simulink model "ex7_pitch"  (R2021b)
settings: Solver=FixedStepAuto  StartTime=0.0  StopTime=120  FixedStep=0.05  RelTol=1e-7
settings Model: Creator=steven  LastModifiedBy=steven

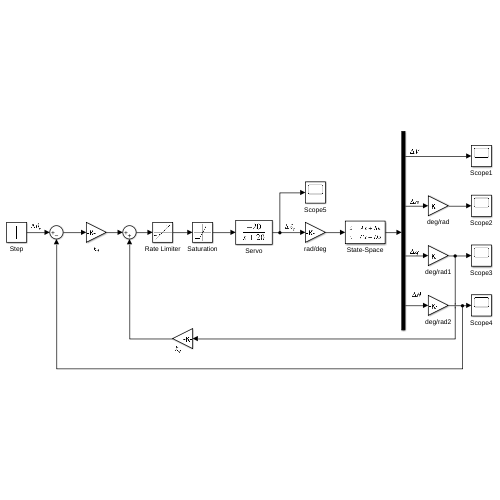
[thumbnail: Simulink's stored preview of the top-level diagram]
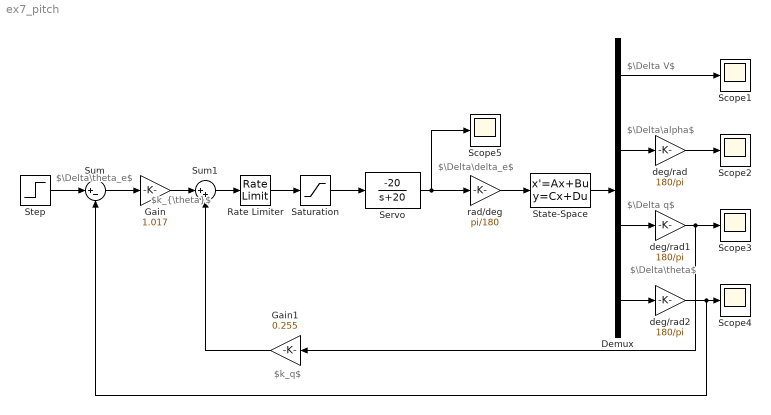
== system ex7_pitch ==
  note: $\Delta\alpha$
  note: $\Delta V$
  note: $\Delta q$
  note: $\Delta\theta$
  note: $\Delta\delta_e$
  note: $\Delta\theta_e$
  note: $k_{\theta}$
  note: $k_q$
  Demux : Demux
  Gain : Gain  Gain=1.017
  Gain1 : Gain  Gain=0.255
  Rate Limiter : RateLimiter  RisingSlewLimit=30  FallingSlewLimit=-30  SampleTimeMode=inherited
  Saturation : Saturate  UpperLimit=15  LowerLimit=-25
  Scope{1..5} (5 alike) : Scope
  Servo : TransferFcn  Numerator=[-20]  Denominator=[1 20]
  State-Space : StateSpace  A=[-0.0045,1.93,0,-9.8; -0.007, -2.02, 1, 0; 0.0062,-6.97,-2.948,0; 0,0,1,0]  B=[0;-0.16;-11.87;0]  C=eye(4)  D=[0;0;0;0]  InitialCondition=0
  Step : Step  Time=0  After=5  SampleTime=0  ZeroCross=off
  Sum : Sum  Inputs=|+-
  Sum1 : Sum  Inputs=|++
  deg/rad : Gain  Gain=180/pi
  deg/rad1 : Gain  Gain=180/pi
  deg/rad2 : Gain  Gain=180/pi
  rad/deg : Gain  Gain=pi/180
  wires:
  Step/1 -> Sum/1
  Saturation/1 -> Servo/1
  Gain/1 -> Sum1/1
  Sum1/1 -> Rate Limiter/1
  Sum/1 -> Gain/1
  Rate Limiter/1 -> Saturation/1
  Servo/1 -> Scope5/1, rad/deg/1
  rad/deg/1 -> State-Space/1
  State-Space/1 -> Demux/1
  Demux/2 -> deg/rad/1
  Demux/3 -> deg/rad1/1
  Demux/4 -> deg/rad2/1
  deg/rad/1 -> Scope2/1
  deg/rad1/1 -> Gain1/1, Scope3/1
  deg/rad2/1 -> Sum/2, Scope4/1
  Demux/1 -> Scope1/1
  Gain1/1 -> Sum1/2
